simulink subsystem "OUTBOUND_MSG_UNMAP"  (R2023a)
settings: Solver=VariableStepAuto  StartTime=0.0  StopTime=10.0  RelTol=1e-3
settings Model: Creator=thesa  LastModifiedBy=thesa

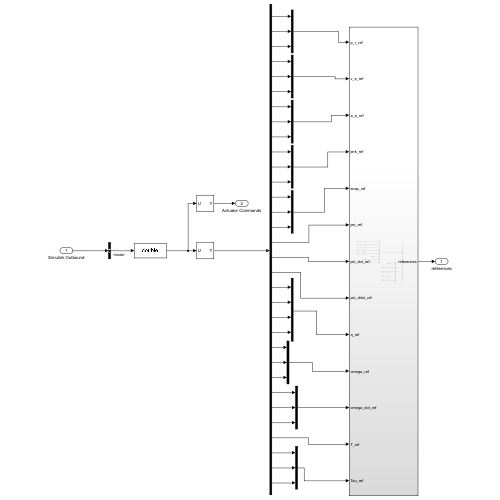
[thumbnail: Simulink's stored preview of the top-level diagram]
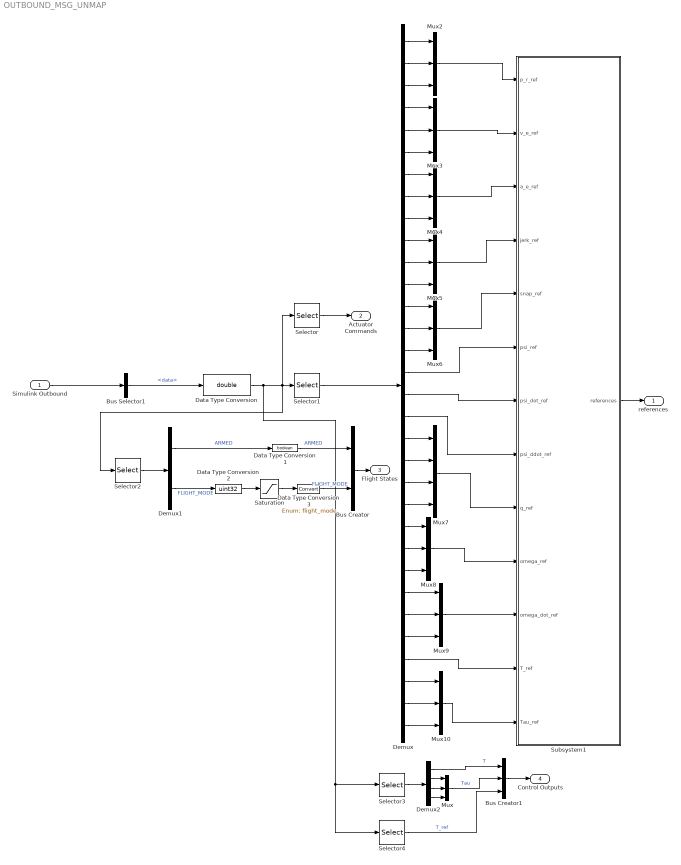
== system OUTBOUND_MSG_UNMAP ==
  Simulink Outbound : Inport
  Bus Creator : BusCreator  Inputs=2
  Bus Creator1 : BusCreator  Inputs=3
  Bus Selector1 : BusSelector  OutputSignals=data
  Data Type Conversion : DataTypeConversion  OutDataTypeStr=double  SaturateOnIntegerOverflow=off  RndMeth=Floor
  Data Type Conversion1 : DataTypeConversion  OutDataTypeStr=boolean  RndMeth=Nearest  SaturateOnIntegerOverflow=off
  Data Type Conversion2 : DataTypeConversion  OutDataTypeStr=uint32  RndMeth=Nearest  SaturateOnIntegerOverflow=off
  Data Type Conversion3 : DataTypeConversion  OutDataTypeStr=Enum: flight_mode  SaturateOnIntegerOverflow=off  RndMeth=Floor
  Demux : Demux  Outputs=32
  Demux1 : Demux  Outputs=2
  Demux2 : Demux
  Mux{,2..6,8..10} (9 alike) : Mux  Inputs=3
  Mux7 : Mux
  Saturation : Saturate  UpperLimit=8  LowerLimit=0
  Selector : Selector  InputPortWidth=58  IndexOptions=Index vector (dialog)  Indices=[1:16]  OutputSizes=1
  Selector1 : Selector  InputPortWidth=58  IndexOptions=Index vector (dialog)  Indices=[(1:32)+16]  OutputSizes=1
  Selector2 : Selector  InputPortWidth=58  IndexOptions=Index vector (dialog)  Indices=[(1:2)+32+16+4]  OutputSizes=1
  Selector3 : Selector  InputPortWidth=58  IndexOptions=Index vector (dialog)  Indices=[(1:4)+16+32]  OutputSizes=1
  Selector4 : Selector  InputPortWidth=58  IndexOptions=Index vector (dialog)  Indices=[(1:3)+32+16+4+2]  OutputSizes=1
  Subsystem1 : Subsystem
  references : Outport
  Actuator Commands : Outport  Port=2
  Flight States : Outport  Port=3
  Control Outputs : Outport  Port=4
  wires:
  Selector/1 -> Actuator Commands/1
  Subsystem1/1(references) -> references/1
  Mux10/1 -> Subsystem1/13(Tau_ref)
  Demux/32 -> Mux10/3
  Demux/30 -> Mux10/1
  Demux/31 -> Mux10/2
  Demux/29 -> Subsystem1/12(T_ref)
  Mux9/1 -> Subsystem1/11(omega_dot_ref)
  Demux/28 -> Mux9/3
  Demux/27 -> Mux9/2
  Demux/26 -> Mux9/1
  Mux8/1 -> Subsystem1/10(omega_ref)
  Demux/24 -> Mux8/2
  Demux/23 -> Mux8/1
  Demux/25 -> Mux8/3
  Mux7/1 -> Subsystem1/9(q_ref)
  Demux/22 -> Mux7/4
  Demux/21 -> Mux7/3
  Demux/20 -> Mux7/2
  Demux/19 -> Mux7/1
  Demux/18 -> Subsystem1/8(psi_ddot_ref)
  Demux/17 -> Subsystem1/7(psi_dot_ref)
  Demux/16 -> Subsystem1/6(psi_ref)
  Mux6/1 -> Subsystem1/5(snap_ref)
  Demux/13 -> Mux6/1
  Demux/14 -> Mux6/2
  Demux/15 -> Mux6/3
  Mux5/1 -> Subsystem1/4(jerk_ref)
  Demux/11 -> Mux5/2
  Demux/12 -> Mux5/3
  Demux/10 -> Mux5/1
  Mux4/1 -> Subsystem1/3(a_e_ref)
  Demux/7 -> Mux4/1
  Demux/9 -> Mux4/3
  Demux/8 -> Mux4/2
  Mux3/1 -> Subsystem1/2(v_e_ref)
  Mux2/1 -> Subsystem1/1(p_r_ref)
  Demux/6 -> Mux3/3
  Demux/4 -> Mux3/1
  Demux/5 -> Mux3/2
  Demux/3 -> Mux2/3
  Demux/1 -> Mux2/1
  Demux/2 -> Mux2/2
  Selector1/1 -> Demux/1
  Data Type Conversion/1 -> Selector2/1, Selector/1, Selector1/1, Selector3/1, Selector4/1
  Bus Selector1/1 -> Data Type Conversion/1  "<data>"
  Simulink Outbound/1 -> Bus Selector1/1
  Selector2/1 -> Demux1/1
  Demux1/1 -> Data Type Conversion1/1  "ARMED"
  Demux1/2 -> Data Type Conversion2/1  "FLIGHT_MODE"
  Bus Creator/1 -> Flight States/1
  Data Type Conversion1/1 -> Bus Creator/1  "ARMED"
  Data Type Conversion2/1 -> Saturation/1
  Data Type Conversion3/1 -> Bus Creator/2  "FLIGHT_MODE"
  Saturation/1 -> Data Type Conversion3/1
  Selector3/1 -> Demux2/1
  Demux2/2 -> Mux/1
  Demux2/3 -> Mux/2
  Demux2/4 -> Mux/3
  Demux2/1 -> Bus Creator1/1  "T"
  Mux/1 -> Bus Creator1/2  "Tau"
  Bus Creator1/1 -> Control Outputs/1
  Selector4/1 -> Bus Creator1/3  "T_ref"

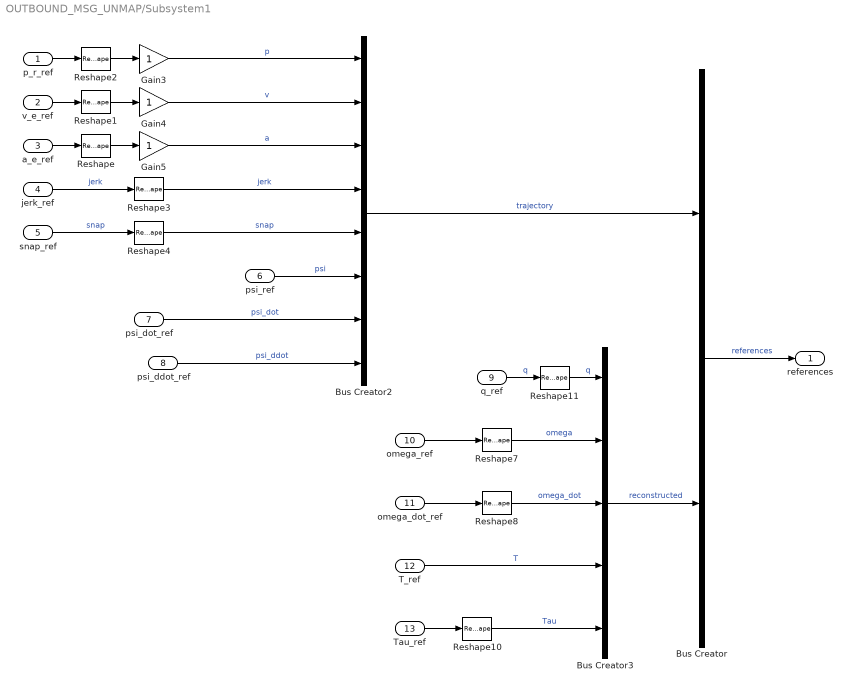
== system OUTBOUND_MSG_UNMAP/Subsystem1 ==
  p_r_ref : Inport
  v_e_ref : Inport  Port=2
  a_e_ref : Inport  Port=3
  jerk_ref : Inport  Port=4
  snap_ref : Inport  Port=5
  psi_ref : Inport  Port=6
  psi_dot_ref : Inport  Port=7
  psi_ddot_ref : Inport  Port=8
  q_ref : Inport  Port=9
  omega_ref : Inport  Port=10
  omega_dot_ref : Inport  Port=11
  T_ref : Inport  Port=12
  Tau_ref : Inport  Port=13
  Bus Creator : BusCreator  Inputs=2
  Bus Creator2 : BusCreator  Inputs=8
  Bus Creator3 : BusCreator  Inputs=5
  Gain3 : Gain
  Gain4 : Gain
  Gain5 : Gain
  Reshape{,1..4,7..8,10} (8 alike) : Reshape  OutputDimensionality=Column vector (2-D)
  Reshape11 : Reshape  OutputDimensionality=Row vector (2-D)
  references : Outport
  wires:
  Reshape10/1 -> Bus Creator3/5  "Tau"
  omega_dot_ref/1 -> Reshape8/1
  Bus Creator2/1 -> Bus Creator/1  "trajectory"
  Bus Creator3/1 -> Bus Creator/2  "reconstructed"
  a_e_ref/1 -> Reshape/1
  v_e_ref/1 -> Reshape1/1
  Reshape11/1 -> Bus Creator3/1  "q"
  Reshape8/1 -> Bus Creator3/3  "omega_dot"
  q_ref/1 -> Reshape11/1  "q"
  Reshape7/1 -> Bus Creator3/2  "omega"
  T_ref/1 -> Bus Creator3/4  "T"
  Bus Creator/1 -> references/1  "references"
  omega_ref/1 -> Reshape7/1
  Tau_ref/1 -> Reshape10/1
  psi_ddot_ref/1 -> Bus Creator2/8  "psi_ddot"
  psi_dot_ref/1 -> Bus Creator2/7  "psi_dot"
  Gain4/1 -> Bus Creator2/2  "v"
  psi_ref/1 -> Bus Creator2/6  "psi"
  snap_ref/1 -> Reshape4/1  "snap"
  jerk_ref/1 -> Reshape3/1  "jerk"
  Gain5/1 -> Bus Creator2/3  "a"
  Gain3/1 -> Bus Creator2/1  "p"
  p_r_ref/1 -> Reshape2/1
  Reshape/1 -> Gain5/1
  Reshape1/1 -> Gain4/1
  Reshape2/1 -> Gain3/1
  Reshape3/1 -> Bus Creator2/4  "jerk"
  Reshape4/1 -> Bus Creator2/5  "snap"
